simulink model "Demo"  (R2024b)
settings: Solver=VariableStepAuto  StartTime=0.0  StopTime=15  FixedStep=0.001  RelTol=1e-3
InitFcn:
  | LCS_parameters
values from neighbouring files (symbols this model uses):
  BREFF = 1.9697    [LCS_parameters.m]
  carMass = 251.54    [LCS_parameters.m]
  CGheight = 0.253    [LCS_parameters.m]
  Cz = 87563    [LCS_parameters.m]
  DREFF = 0.54832    [LCS_parameters.m]
  FNOMIN = 1295    [LCS_parameters.m]
  FREFF = 0.017609    [LCS_parameters.m]
  gearRatio = 13.75    [LCS_parameters.m]
  LONGVL = 10    [LCS_parameters.m]
  maxTorque = 21    [LCS_parameters.m]
  nominalWheelRadius = 0.197    [LCS_parameters.m]
  optimalSlipRatio = 0.11    [LCS_parameters.m]
  Q_REO = 1    [LCS_parameters.m]
  Q_V1 = 0.0034187    [LCS_parameters.m]
  ss_error = [88.7600822305642	89.0376071734511	89.3159282635258	89.5955216735338	89.8756411218665	90.1570974487717	90.4395677327939	90.7230274541677	91.0072189085757	91.2921635447457	91.5779490537006	91.8650704841512	92.1538219996540	92.4426633861175	92.7316475908439	93.0233476422096	93.3140548464672	93.6068138765075	93.9008352694172	94.1935963586418	94.4902272246880	94.7850545124692	95.0823324329676	95.38056 ...(+2780 chars)    [LCS_parameters.m]
  unloadedRadius = 0.2032    [LCS_parameters.m]
  wheelbaseLength = 1.53    [LCS_parameters.m]
undefined symbols (not defined in the file or in its folder): dspblkCoreblockFVToolHelper, gcbh
libraries: simulink x3, SignalEditorBlockLib x2, Solver_SF x1
settings Model: Creator=account  LastModifiedBy=xoxi.1

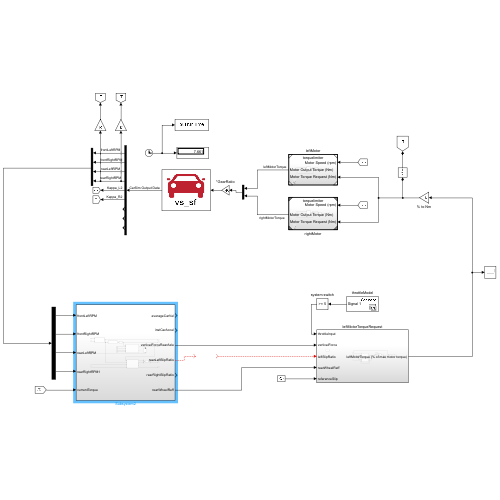
[thumbnail: Simulink's stored preview of the top-level diagram]
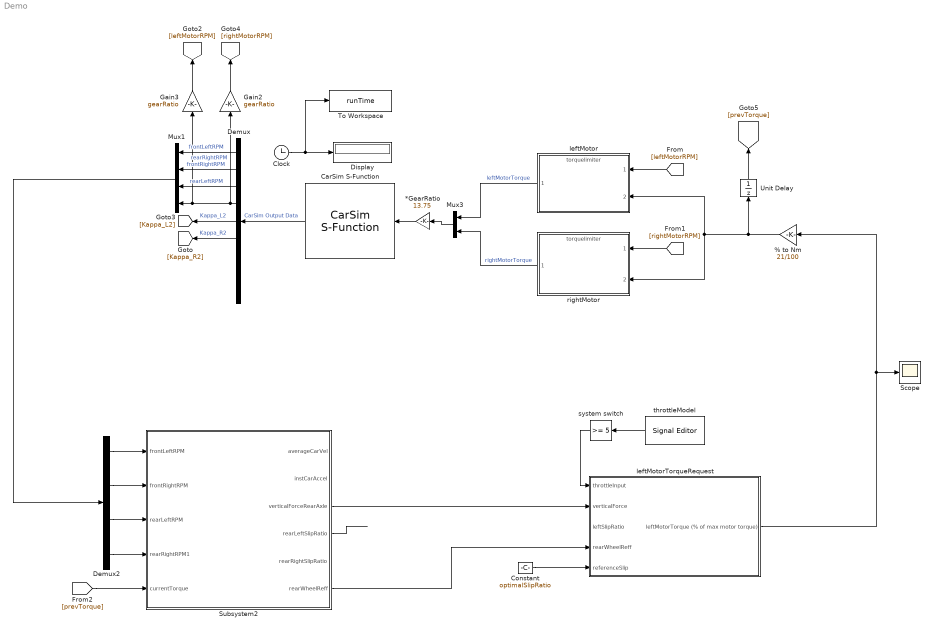
== system Demo ==
  % to Nm : Gain  Gain=21/100
  *GearRatio : Gain  Gain=13.75
  CarSim S-Function : Solver_SF/CarSim S-Function  Priority=1  SIMFILE=simfile.sim  Run_RTs=off  vs_state_ind=Run  StopMode_ind=Vehicle Model
  Clock : Clock
  Constant : Constant  Value=optimalSlipRatio
  Demux : Demux  Outputs=9
  Demux2 : Demux
  Display : Display
  Gain2 : Gain  Gain=gearRatio
  Gain3 : Gain  Gain=gearRatio
  Mux1 : Mux
  Mux3 : Mux  Inputs=2
  Scope : Scope
  Subsystem2 : Subsystem
  To Workspace : ToWorkspace  VariableName=runTime  SaveFormat=Timeseries  SampleTime=-1
  Unit Delay : UnitDelay  SampleTime=-1  HasFrameUpgradeWarning=on
  leftMotor : ModelReference  ModelNameDialog=torquelimiter.slx  SimulationMode=Normal  ModelReferenceVersion=1.5
  leftMotorTorqueRequest : Subsystem
  rightMotor : ModelReference  ModelNameDialog=torquelimiter.slx  SimulationMode=Normal  ModelReferenceVersion=1.5
  system switch : simulink/Logic and Bit Operations/Compare To Constant  relop=>=  const=5  OutDataTypeStr=boolean
  throttleModel : SignalEditorBlockLib/Signal Editor  FileName=throttleModel.mat  ActiveScenario=Scenario  ActiveSignal=Signal 1  IsBus=off  OutputBusObjectStr=Bus: BusObject  SampleTime=0  ZeroCross=off  OutputAfterFinalValue=Setting to zero  Unit=inherit  PreserveSignalName=on  ApplySigPropsToAllScenarios=on  ApplySigPropsToAllSignals=off
  wires:
  CarSim S-Function/1 -> Demux/1  "CarSim Output Data"
  Demux/1 -> Mux1/1  "frontLeftRPM"
  Demux/2 -> Mux1/2  "frontRightRPM"
  Demux/3 -> Mux1/3  "rearLeftRPM"
  Mux1/1 -> Demux2/1
  Clock/1 -> To Workspace/1, Display/1
  leftMotor/1 -> Mux3/1  "leftMotorTorque"
  rightMotor/1 -> Mux3/2  "rightMotorTorque"
  Demux/4 -> Gain2/1, Mux1/4, Gain3/1  "rearRightRPM"
  [rightMotorRPM] -> rightMotor/1
  [leftMotorRPM] -> leftMotor/1
  Demux/5 -> [Kappa_L2]  "Kappa_L2"
  Demux/6 -> [Kappa_R2]  "Kappa_R2"
  % to Nm/1 -> Unit Delay/1, rightMotor/2, leftMotor/2
  *GearRatio/1 -> CarSim S-Function/1
  Mux3/1 -> *GearRatio/1
  Gain3/1 -> [leftMotorRPM]
  Gain2/1 -> [rightMotorRPM]
  Demux2/1 -> Subsystem2/1(frontLeftRPM)
  Demux2/2 -> Subsystem2/2(frontRightRPM)
  [prevTorque] -> Subsystem2/5(currentTorque)
  Demux2/4 -> Subsystem2/4(rearRightRPM1)
  Demux2/3 -> Subsystem2/3(rearLeftRPM)
  Unit Delay/1 -> [prevTorque]
  Constant/1 -> leftMotorTorqueRequest/5(referenceSlip)
  Subsystem2/6(rearWheelReff) -> leftMotorTorqueRequest/4(rearWheelReff)
  Subsystem2/4(rearLeftSlipRatio) -> ?
  throttleModel/1 -> system switch/1
  system switch/1 -> leftMotorTorqueRequest/1(throttleInput)
  leftMotorTorqueRequest/1(leftMotorTorque (% of max motor torque)) -> % to Nm/1, Scope/1
  Subsystem2/3(verticalForceRearAxle) -> leftMotorTorqueRequest/2(verticalForce)
  ? -> leftMotorTorqueRequest/3(leftSlipRatio)

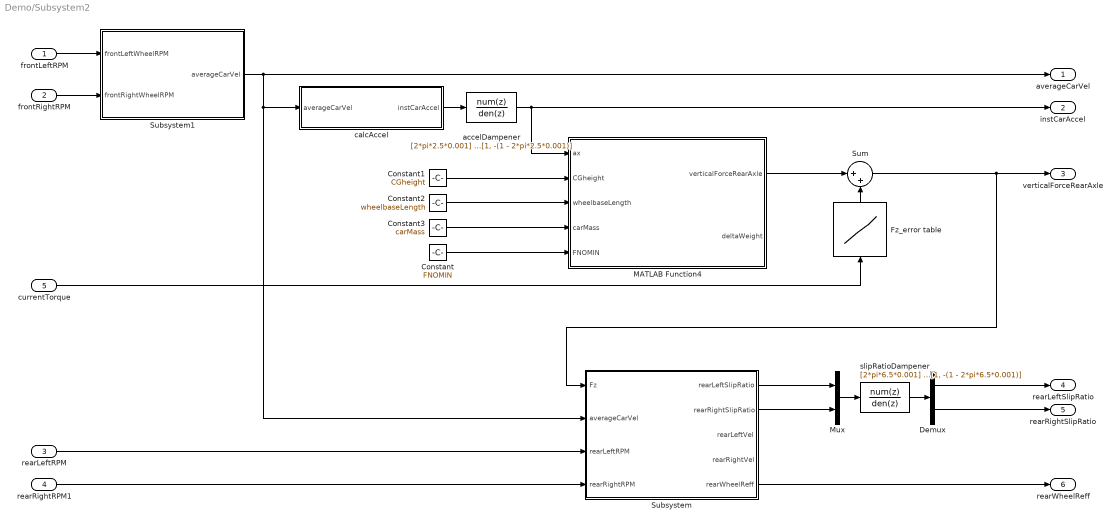
== system Demo/Subsystem2 ==
  frontLeftRPM : Inport
  frontRightRPM : Inport  Port=2
  rearLeftRPM : Inport  Port=3
  rearRightRPM1 : Inport  Port=4
  currentTorque : Inport  Port=5
  Constant : Constant  Value=FNOMIN
  Constant1 : Constant  Value=CGheight
  Constant2 : Constant  Value=wheelbaseLength
  Constant3 : Constant  Value=carMass
  Demux : Demux  Outputs=2
  Fz_error table : Lookup_n-D  NumberOfTableDimensions=1  BreakpointsForDimension1=[7:0.5:100]  Table=ss_error  InternalRulePriority=Speed  RndMeth=Simplest
  MATLAB Function4 : MATLAB Function  TreatAsAtomicUnit=on
  Mux : Mux  Inputs=2
  Subsystem : Subsystem
  Subsystem1 : Subsystem
  Sum : Sum  Inputs=|++
  accelDampener : DiscreteTransferFcn  LoadFcn=dspblkCoreblockFVToolHelper(gcbh,'load');  Numerator=[2*pi*2.5*0.001]  Denominator=[1, -(1 - 2*pi*2.5*0.001)]
      settings: CopyFcn=dspblkCoreblockFVToolHelper(gcbh,'copy');  DeleteFcn=dspblkCoreblockFVToolHelper(gcbh,'close');  ModelCloseFcn=dspblkCoreblockFVToolHelper(gcbh,'close');  PreSaveFcn=dspblkCoreblockFVToolHelper(gcbh,'presave');  PostSaveFcn=dspblkCoreblockFVToolHelper(gcbh,'postsave');  CloseFcn=dspblkCoreblockFVToolHelper(gcbh,'close');
  calcAccel : Subsystem
  slipRatioDampener : DiscreteTransferFcn  LoadFcn=dspblkCoreblockFVToolHelper(gcbh,'load');  Numerator=[2*pi*6.5*0.001]  Denominator=[1, -(1 - 2*pi*6.5*0.001)]
      settings: CopyFcn=dspblkCoreblockFVToolHelper(gcbh,'copy');  DeleteFcn=dspblkCoreblockFVToolHelper(gcbh,'close');  ModelCloseFcn=dspblkCoreblockFVToolHelper(gcbh,'close');  PreSaveFcn=dspblkCoreblockFVToolHelper(gcbh,'presave');  PostSaveFcn=dspblkCoreblockFVToolHelper(gcbh,'postsave');  CloseFcn=dspblkCoreblockFVToolHelper(gcbh,'close');
  averageCarVel : Outport
  instCarAccel : Outport  Port=2
  verticalForceRearAxle : Outport  Port=3
  rearLeftSlipRatio : Outport  Port=4
  rearRightSlipRatio : Outport  Port=5
  rearWheelReff : Outport  Port=6
  wires:
  frontLeftRPM/1 -> Subsystem1/1(frontLeftWheelRPM)
  Subsystem1/1(averageCarVel) -> averageCarVel/1, Subsystem/2(averageCarVel), calcAccel/1(averageCarVel)
  calcAccel/1(instCarAccel) -> accelDampener/1
  frontRightRPM/1 -> Subsystem1/2(frontRightWheelRPM)
  Constant3/1 -> MATLAB Function4/4(carMass)
  Constant1/1 -> MATLAB Function4/2(CGheight)
  Constant2/1 -> MATLAB Function4/3(wheelbaseLength)
  accelDampener/1 -> instCarAccel/1, MATLAB Function4/1(ax)
  currentTorque/1 -> Fz_error table/1
  Sum/1 -> Subsystem/1(Fz), verticalForceRearAxle/1
  Fz_error table/1 -> Sum/2
  Constant/1 -> MATLAB Function4/5(FNOMIN)
  rearLeftRPM/1 -> Subsystem/3(rearLeftRPM)
  rearRightRPM1/1 -> Subsystem/4(rearRightRPM)
  Subsystem/1(rearLeftSlipRatio) -> Mux/1
  Subsystem/2(rearRightSlipRatio) -> Mux/2
  Subsystem/5(rearWheelReff) -> rearWheelReff/1
  MATLAB Function4/1(verticalForceRearAxle) -> Sum/1
  Mux/1 -> slipRatioDampener/1
  slipRatioDampener/1 -> Demux/1
  Demux/2 -> rearRightSlipRatio/1
  Demux/1 -> rearLeftSlipRatio/1

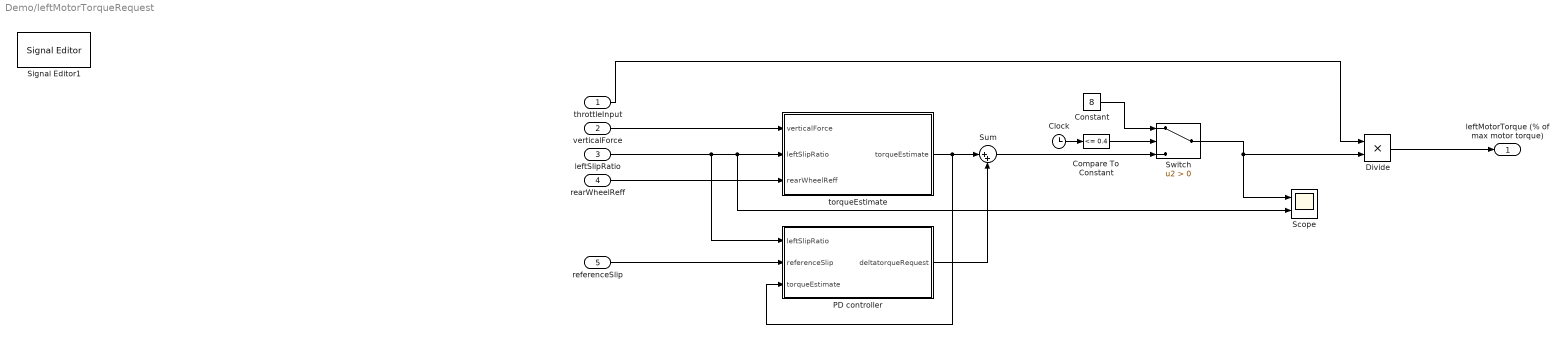
== system Demo/leftMotorTorqueRequest ==
  throttleInput : Inport
  verticalForce : Inport  Port=2
  leftSlipRatio : Inport  Port=3
  rearWheelReff : Inport  Port=4
  referenceSlip : Inport  Port=5
  Clock : Clock
  Compare To Constant : simulink/Logic and Bit Operations/Compare To Constant  relop=<=  const=0.4  OutDataTypeStr=boolean
  Constant : Constant  Value=8
  Divide : Product  Inputs=**
  PD controller : Subsystem
  Scope : Scope  NumInputPorts=2
  Signal Editor1 : SignalEditorBlockLib/Signal Editor  FileName=bullshit2.mat  ActiveScenario=Scenario  ActiveSignal=Signal 1  IsBus=off  OutputBusObjectStr=Bus: BusObject  SampleTime=0  ZeroCross=off  OutputAfterFinalValue=Setting to zero  Unit=inherit  PreserveSignalName=on  ApplySigPropsToAllScenarios=on  ApplySigPropsToAllSignals=off
  Sum : Sum  Inputs=|++
  Switch : Switch  Criteria=u2 > Threshold  SaturateOnIntegerOverflow=off  InputSameDT=off
  torqueEstimate : Subsystem
  leftMotorTorque (% of max motor torque) : Outport
  wires:
  verticalForce/1 -> torqueEstimate/1(verticalForce)
  PD controller/1(deltatorqueRequest) -> Sum/2
  torqueEstimate/1(torqueEstimate) -> PD controller/3(torqueEstimate), Sum/1
  leftSlipRatio/1 -> PD controller/1(leftSlipRatio), Scope/2, torqueEstimate/2(leftSlipRatio)
  referenceSlip/1 -> PD controller/2(referenceSlip)
  rearWheelReff/1 -> torqueEstimate/3(rearWheelReff)
  Divide/1 -> leftMotorTorque (% of max motor torque)/1
  throttleInput/1 -> Divide/1
  Clock/1 -> Compare To Constant/1
  Compare To Constant/1 -> Switch/2
  Sum/1 -> Switch/3
  Switch/1 -> Scope/1, Divide/2
  Constant/1 -> Switch/1

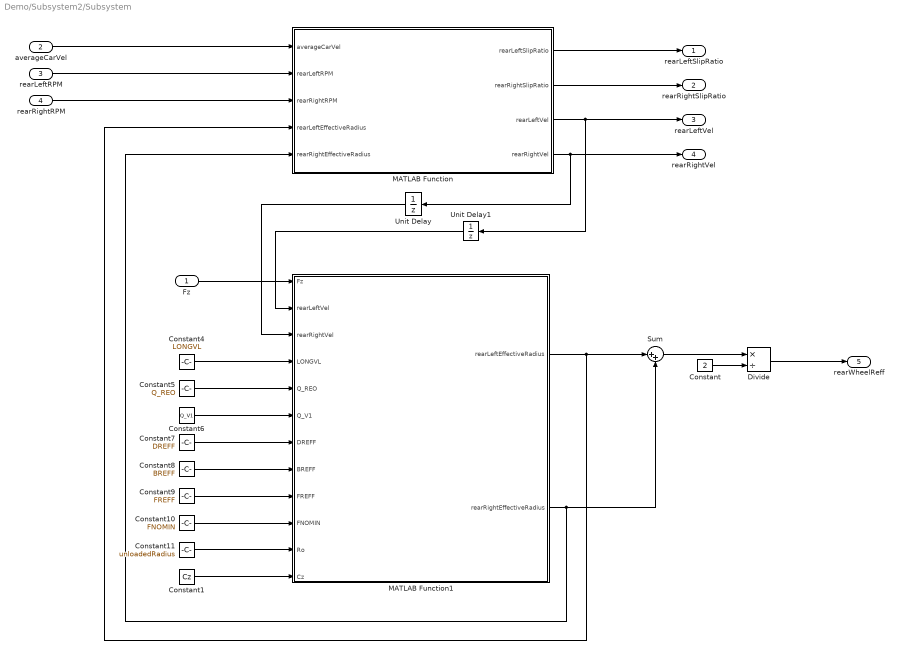
== system Demo/Subsystem2/Subsystem ==
  Fz : Inport
  averageCarVel : Inport  Port=2
  rearLeftRPM : Inport  Port=3
  rearRightRPM : Inport  Port=4
  Constant : Constant  Value=2
  Constant1 : Constant  Value=Cz
  Constant10 : Constant  Value=FNOMIN
  Constant11 : Constant  Value=unloadedRadius
  Constant4 : Constant  Value=LONGVL
  Constant5 : Constant  Value=Q_REO
  Constant6 : Constant  Value=Q_V1
  Constant7 : Constant  Value=DREFF
  Constant8 : Constant  Value=BREFF
  Constant9 : Constant  Value=FREFF
  Divide : Product  Inputs=*/
  MATLAB Function : MATLAB Function  TreatAsAtomicUnit=on
  MATLAB Function1 : MATLAB Function  TreatAsAtomicUnit=on
  Sum : Sum  Inputs=|++
  Unit Delay : UnitDelay  SampleTime=-1  HasFrameUpgradeWarning=on
  Unit Delay1 : UnitDelay  SampleTime=-1  HasFrameUpgradeWarning=on
  rearLeftSlipRatio : Outport
  rearRightSlipRatio : Outport  Port=2
  rearLeftVel : Outport  Port=3
  rearRightVel : Outport  Port=4
  rearWheelReff : Outport  Port=5
  wires:
  Constant8/1 -> MATLAB Function1/8(BREFF)
  MATLAB Function/3(rearLeftVel) -> rearLeftVel/1, Unit Delay1/1
  averageCarVel/1 -> MATLAB Function/1(averageCarVel)
  Unit Delay/1 -> MATLAB Function1/3(rearRightVel)
  Constant4/1 -> MATLAB Function1/4(LONGVL)
  Constant6/1 -> MATLAB Function1/6(Q_V1)
  Constant9/1 -> MATLAB Function1/9(FREFF)
  MATLAB Function1/2(rearRightEffectiveRadius) -> Sum/2, MATLAB Function/5(rearRightEffectiveRadius)
  MATLAB Function/4(rearRightVel) -> rearRightVel/1, Unit Delay/1
  Constant5/1 -> MATLAB Function1/5(Q_REO)
  Fz/1 -> MATLAB Function1/1(Fz)
  Unit Delay1/1 -> MATLAB Function1/2(rearLeftVel)
  Constant7/1 -> MATLAB Function1/7(DREFF)
  Constant10/1 -> MATLAB Function1/10(FNOMIN)
  Constant11/1 -> MATLAB Function1/11(Ro)
  rearLeftRPM/1 -> MATLAB Function/2(rearLeftRPM)
  rearRightRPM/1 -> MATLAB Function/3(rearRightRPM)
  MATLAB Function/2(rearRightSlipRatio) -> rearRightSlipRatio/1
  MATLAB Function/1(rearLeftSlipRatio) -> rearLeftSlipRatio/1
  MATLAB Function1/1(rearLeftEffectiveRadius) -> Sum/1, MATLAB Function/4(rearLeftEffectiveRadius)
  Constant1/1 -> MATLAB Function1/12(Cz)
  Sum/1 -> Divide/1
  Constant/1 -> Divide/2
  Divide/1 -> rearWheelReff/1

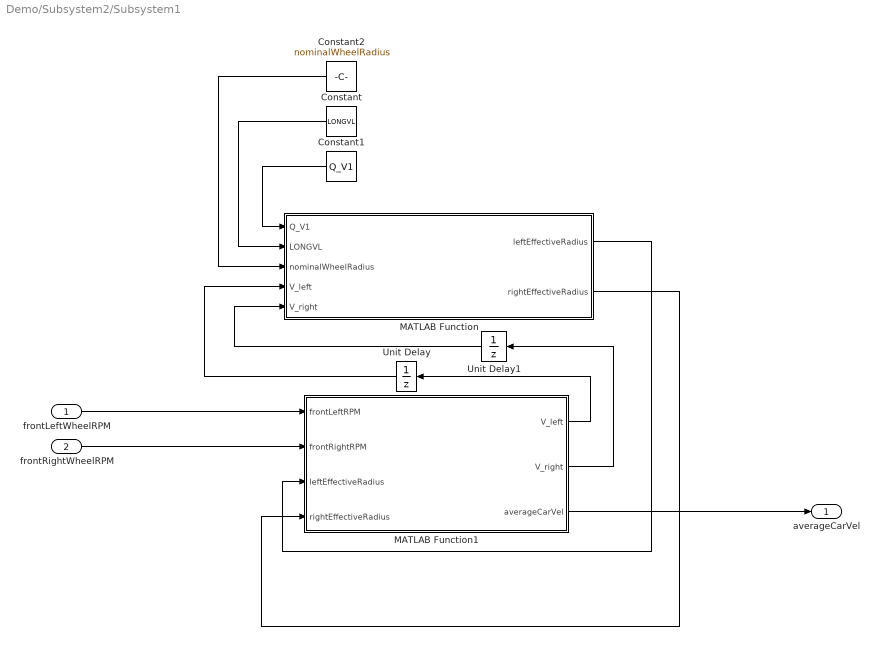
== system Demo/Subsystem2/Subsystem1 ==
  frontLeftWheelRPM : Inport
  frontRightWheelRPM : Inport  Port=2
  Constant : Constant  Value=LONGVL
  Constant1 : Constant  Value=Q_V1
  Constant2 : Constant  Value=nominalWheelRadius
  MATLAB Function : MATLAB Function  TreatAsAtomicUnit=on
  MATLAB Function1 : MATLAB Function  TreatAsAtomicUnit=on
  Unit Delay : UnitDelay  SampleTime=-1  HasFrameUpgradeWarning=on
  Unit Delay1 : UnitDelay  SampleTime=-1  HasFrameUpgradeWarning=on
  averageCarVel : Outport
  wires:
  frontLeftWheelRPM/1 -> MATLAB Function1/1(frontLeftRPM)
  frontRightWheelRPM/1 -> MATLAB Function1/2(frontRightRPM)
  MATLAB Function1/3(averageCarVel) -> averageCarVel/1
  Constant1/1 -> MATLAB Function/1(Q_V1)
  Constant/1 -> MATLAB Function/2(LONGVL)
  Constant2/1 -> MATLAB Function/3(nominalWheelRadius)
  MATLAB Function1/1(V_left) -> Unit Delay/1
  MATLAB Function1/2(V_right) -> Unit Delay1/1
  Unit Delay/1 -> MATLAB Function/4(V_left)
  Unit Delay1/1 -> MATLAB Function/5(V_right)
  MATLAB Function/1(leftEffectiveRadius) -> MATLAB Function1/3(leftEffectiveRadius)
  MATLAB Function/2(rightEffectiveRadius) -> MATLAB Function1/4(rightEffectiveRadius)

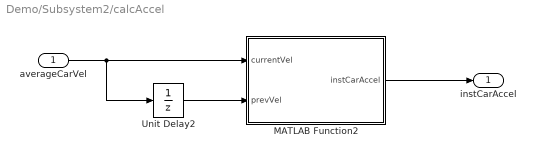
== system Demo/Subsystem2/calcAccel ==
  averageCarVel : Inport
  MATLAB Function2 : MATLAB Function  TreatAsAtomicUnit=on
  Unit Delay2 : UnitDelay  SampleTime=-1  HasFrameUpgradeWarning=on
  instCarAccel : Outport
  wires:
  Unit Delay2/1 -> MATLAB Function2/2(prevVel)
  MATLAB Function2/1(instCarAccel) -> instCarAccel/1
  averageCarVel/1 -> MATLAB Function2/1(currentVel), Unit Delay2/1

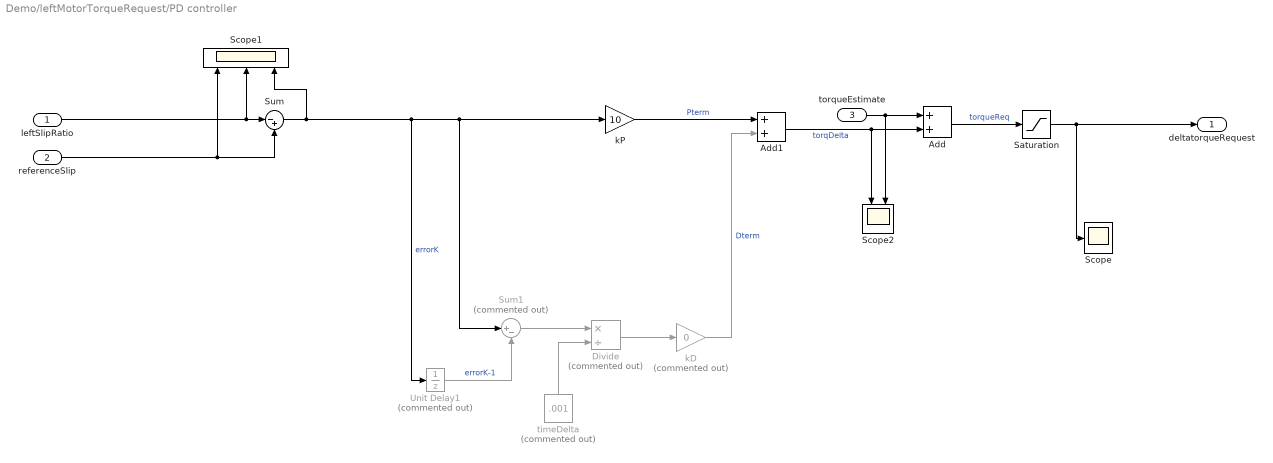
== system Demo/leftMotorTorqueRequest/PD controller ==
  leftSlipRatio : Inport
  referenceSlip : Inport  Port=2
  torqueEstimate : Inport  Port=3
  Add : Sum
  Add1 : Sum
  Divide : Product  Commented=on  Inputs=*/
  Saturation : Saturate  UpperLimit=100  LowerLimit=0
  Scope : Scope
  Scope1 : Scope  NumInputPorts=3
  Scope2 : Scope  NumInputPorts=2
  Sum : Sum  Inputs=|-+
  Sum1 : Sum  Commented=on  Inputs=|+-
  Unit Delay1 : UnitDelay  Commented=on  SampleTime=-1  HasFrameUpgradeWarning=on
  kD : Gain  Commented=on  Gain=0
  kP : Gain  Gain=10
  timeDelta : Constant  Commented=on  Value=.001
  deltatorqueRequest : Outport
  wires:
  Saturation/1 -> Scope/1, deltatorqueRequest/1
  Add1/1 -> Add/2, Scope2/1  "torqDelta"
  leftSlipRatio/1 -> Sum/1, Scope1/2
  Divide/1 -> kD/1
  kD/1 -> Add1/2  "Dterm"
  Add/1 -> Saturation/1  "torqueReq"
  Unit Delay1/1 -> Sum1/2  "errorK-1"
  Sum1/1 -> Divide/1
  kP/1 -> Add1/1  "Pterm"
  Sum/1 -> kP/1, Sum1/1, Unit Delay1/1, Scope1/3  "errorK"
  timeDelta/1 -> Divide/2
  referenceSlip/1 -> Sum/2, Scope1/1
  torqueEstimate/1 -> Add/1, Scope2/2

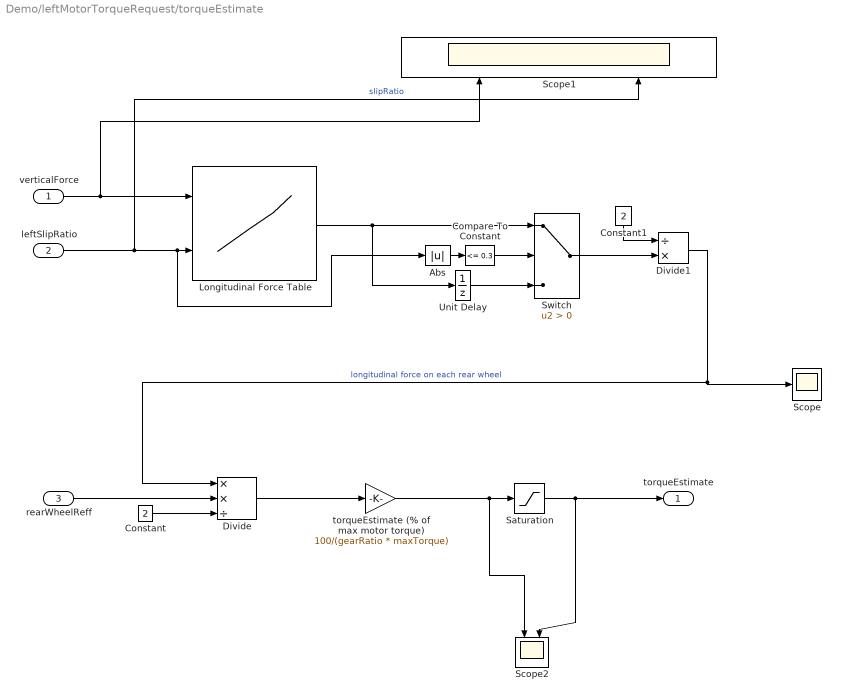
== system Demo/leftMotorTorqueRequest/torqueEstimate ==
  verticalForce : Inport
  leftSlipRatio : Inport  Port=2
  rearWheelReff : Inport  Port=3
  Abs : Abs  SaturateOnIntegerOverflow=off
  Compare To Constant : simulink/Logic and Bit Operations/Compare To Constant  relop=<=  const=0.3  OutDataTypeStr=boolean
  Constant : Constant  Value=2
  Constant1 : Constant  Value=2
  Divide : Product  Inputs=**/
  Divide1 : Product  Inputs=/*
  Longitudinal Force Table : Lookup_n-D  BreakpointsForDimension1=[200 400 600 800 1000 1200 1400 1600 1800 2000]  BreakpointsForDimension2=[-0.020, -0.010, 0.000, 0.010, 0.020, 0.030, 0.040, 0.050, 0.060, 0.070, 0.080, 0.090, 0.100, 0.110, 0.120, 0.130, 0.140, 0.150, 0.160, 0.170, 0.180, 0.190, 0.200]  BreakpointsForDimension3=[5, 7]  Table=|  InternalRulePriority=Speed  RndMeth=Simplest
      | [
      | -189.59  -97.79   0.00   97.79   189.59   270.69   338.40   392.01   432.37   461.20   480.52   492.30   498.31   500.00   498.51   494.76   489.41   482.98   475.85   468.31   460.55   452.74   444.96
      | -379.18  -195.58  0.00   195.58  379.18   541.39   676.79   784.02   864.75   922.40   961.03   984.61   996.63   1000.00  997.03   989.51   978.81   965.96   951.70   936.62   921.11   905.47   889.92
      | -568.78  -293.37  0.00   293.37  568.78   812.08   1015.19  1176.03  1297.12  1383.60  1441.55  1476.91  1494.94  1500.00  1495.54  1484.27  1468.22  1448.93  1427.56  1404.93  1381.66  1358.21  1334.88
      | -758.37  -391.16  0.00   391.16  758.37   1082.78  1353.58  1568.04  1729.50  1844.80  1922.07  1969.22  1993.26  2000.00  1994.06  1979.02  1957.62  1931.91  1903.41  1873.24  1842.22  1810.95  1779.85
      | -947.96  -488.95  0.00   488.95  947.96   1353.47  1691.98  1960.05  2161.87  2306.00  2402.58  2461.52  2491.57  2500.00  2492.57  2473.78  2447.03  2414.89  2379.26  2341.55  2302.77  2263.68  2224.81
      | -1137.55 -586.74  0.00   586.74  1137.55  1624.17  2030.37  2352.06  2594.25  2767.21  2883.10  2953.83  2989.89  3000.00  2991.08  2968.53  2936.43  2897.87  2855.11  2809.85  2763.33  2716.42  2669.77
      | -1327.14 -684.53  0.00   684.53  1327.14  1894.86  2368.77  2744.07  3026.62  3228.41  3363.61  3446.13  3488.20  3499.99  3489.60  3463.29  3425.84  3380.84  3330.96  3278.16  3223.88  3169.16  3114.73
      | -1516.74 -782.32  0.00   782.32  1516.74  2165.56  2707.16  3136.08  3459.00  3689.61  3844.13  3938.43  3986.52  3999.99  3988.11  3958.04  3915.25  3863.82  3806.81  3746.47  3684.44  3621.89  3559.69
      | -1706.33 -880.11  0.00   880.11  1706.33  2436.25  3045.56  3528.08  3891.37  4150.81  4324.65  4430.74  4484.83  4499.99  4486.63  4452.80  4404.65  4346.80  4282.67  4214.78  4144.99  4074.63  4004.65
      | -1895.92 -977.90  0.00   977.90  1895.92  2706.95  3383.95  3920.09  4323.75  4612.01  4805.16  4923.04  4983.15  4999.99  4985.14  4947.55  4894.06  4829.78  4758.52  4683.09  4605.54  4527.36  4449.62
      | ]
      settings: InputPortMap=u0,u1
  Saturation : Saturate  UpperLimit=100  LowerLimit=0
  Scope : Scope
  Scope1 : Scope  NumInputPorts=2
  Scope2 : Scope  NumInputPorts=2
  Switch : Switch  Criteria=u2 > Threshold  SaturateOnIntegerOverflow=off  InputSameDT=off
  Unit Delay : UnitDelay  SampleTime=-1  HasFrameUpgradeWarning=on
  torqueEstimate (% of max motor torque) : Gain  Gain=100/(gearRatio * maxTorque)
  torqueEstimate : Outport
  wires:
  Divide/1 -> torqueEstimate (% of max motor torque)/1
  torqueEstimate (% of max motor torque)/1 -> Scope2/1, Saturation/1
  leftSlipRatio/1 -> Abs/1, Longitudinal Force Table/2, Scope1/2  "slipRatio"
  rearWheelReff/1 -> Divide/2
  Divide1/1 -> Scope/1, Divide/1  "longitudinal force on each rear wheel"
  Constant/1 -> Divide/3
  Saturation/1 -> Scope2/2, torqueEstimate/1
  Longitudinal Force Table/1 -> Unit Delay/1, Switch/1
  Constant1/1 -> Divide1/1
  Abs/1 -> Compare To Constant/1
  Compare To Constant/1 -> Switch/2
  Switch/1 -> Divide1/2
  verticalForce/1 -> Scope1/1, Longitudinal Force Table/1
  Unit Delay/1 -> Switch/3

== matlab function Demo/Subsystem2/calcAccel/MATLAB Function2 ==
  data: currentVel input; instCarAccel output; prevVel input
function instCarAccel = calcInstaAccel(currentVel, prevVel)

instCarAccel = (currentVel - prevVel)/0.001;

instCarAccel = instCarAccel;

end

== matlab function Demo/Subsystem2/Subsystem1/MATLAB Function ==
  data: Q_V1 input; leftEffectiveRadius output; LONGVL input; nominalWheelRadius input; V_left input; rightEffectiveRadius output; V_right input
function [leftEffectiveRadius, rightEffectiveRadius] = calculateEffectiveRadius(Q_V1, LONGVL, nominalWheelRadius, V_left, V_right)

leftEffectiveRadius = nominalWheelRadius * (1 + Q_V1 * (V_left / LONGVL)^2);
rightEffectiveRadius = nominalWheelRadius * (1 + Q_V1 * (V_right / LONGVL)^2);

end

== matlab function Demo/Subsystem2/Subsystem1/MATLAB Function1 ==
  data: V_left output; V_right output; frontLeftRPM input; averageCarVel output; frontRightRPM input; leftEffectiveRadius input; rightEffectiveRadius input
function [V_left, V_right, averageCarVel] = caclVelwithRealRe(frontLeftRPM, frontRightRPM, leftEffectiveRadius, rightEffectiveRadius)

V_left = leftEffectiveRadius * (frontLeftRPM * 2*pi/60);
V_right = rightEffectiveRadius * (frontRightRPM * 2*pi/60);

averageCarVel = (V_left+V_right)/2;

end

== matlab function Demo/Subsystem2/MATLAB Function4 ==
  data: ax input; CGheight input; wheelbaseLength input; carMass input; verticalForceRearAxle output; deltaWeight output; FNOMIN input
function [verticalForceRearAxle, deltaWeight] = calcVerticalForce(ax, CGheight, wheelbaseLength, carMass, FNOMIN)

deltaWeight = (carMass * ax * CGheight) / wheelbaseLength;

verticalForceRearAxle = FNOMIN + deltaWeight;

end

== matlab function Demo/Subsystem2/Subsystem/MATLAB Function ==
  data: rearLeftSlipRatio output; rearRightSlipRatio output; averageCarVel input; rearLeftRPM input; rearLeftVel output; rearRightRPM input; rearLeftEffectiveRadius input; rearRightEffectiveRadius input; rearRightVel output
function [rearLeftSlipRatio, rearRightSlipRatio, rearLeftVel, rearRightVel] = calculateRearVel(averageCarVel, rearLeftRPM, rearRightRPM, rearLeftEffectiveRadius, rearRightEffectiveRadius)

rearLeftVel = rearLeftEffectiveRadius * (rearLeftRPM * 2*pi/60);
rearRightVel = rearRightEffectiveRadius * (rearRightRPM * 2*pi/60);

rearLeftSlipRatio = (rearLeftVel/averageCarVel) - 1 -0.005;
rearRightSlipRatio = (rearRightVel/averageCarVel) - 1 - 0.005;
end

== matlab function Demo/Subsystem2/Subsystem/MATLAB Function1 ==
  data: Fz input; rearLeftVel input; rearLeftEffectiveRadius output; rearRightVel input; LONGVL input; Q_REO input; Q_V1 input; DREFF input; BREFF input; FREFF input; FNOMIN input; Ro input; rearRightEffectiveRadius output; Cz input
function [rearLeftEffectiveRadius, rearRightEffectiveRadius] = calculateRearEffectiveRadius(Fz, rearLeftVel, rearRightVel, LONGVL, Q_REO, Q_V1, DREFF, BREFF, FREFF, FNOMIN, Ro, Cz)
    
    Fz = Fz / 2;  % split total axle load equally per wheel
    
    rearLeftRomega  = Ro * (Q_REO + Q_V1 * (rearLeftVel  / LONGVL)^2);
    rearRightRomega = Ro * (Q_REO + Q_V1 * (rearRightVel / LONGVL)^2);
    
    rearLeftEffectiveRadius  = rearLeftRomega  - (Fz / Cz) * (DREFF * atan(BREFF * Fz / FNOMIN) + FREFF * Fz / FNOMIN);
    rearRightEffectiveRadius = rearRightRomega - (Fz / Cz) * (DREFF * atan(BREFF * Fz / FNOMIN) + FREFF * Fz / FNOMIN);

    rearLeftEffectiveRadius = rearLeftEffectiveRadius - 0.0023;
    rearRightEffectiveRadius = rearRightEffectiveRadius - 0.0023;

end
